simulink model "kyvadlo"  (R2017b)
settings: Solver=ode45  StartTime=0.0  StopTime=30  MaxStep=0.015  RelTol=1e-3
settings Model: Creator=ladislav  LastModifiedBy=ladislav

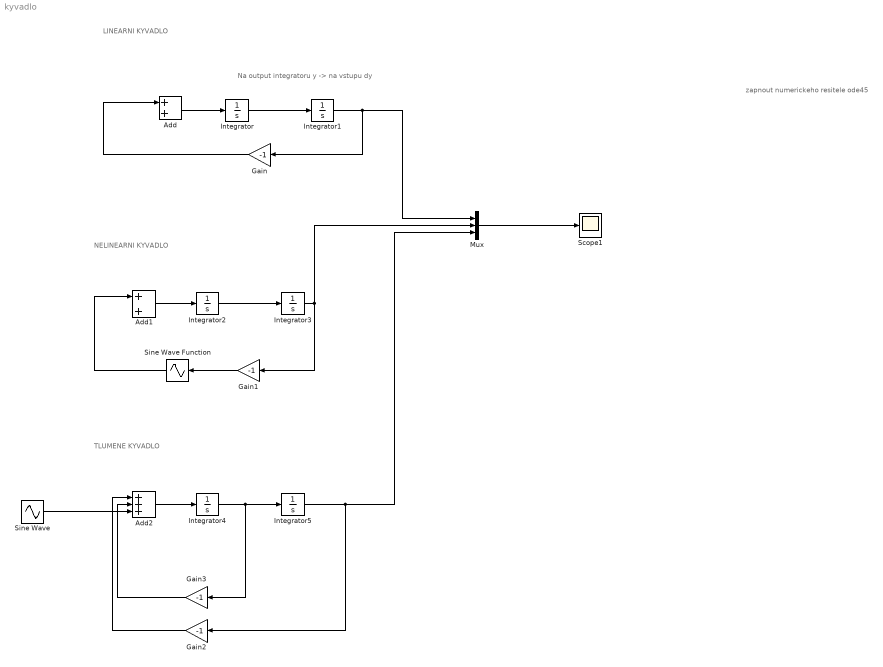
== system kyvadlo ==
  note: zapnout numerickeho resitele ode45
  note: LINEARNI KYVADLO
  note: Na output integratoru y -> na vstupu dy
  note: NELINEARNI KYVADLO
  note: TLUMENE KYVADLO
  Add : Sum
  Add1 : Sum
  Add2 : Sum  Inputs=+++
  Gain{,1..3} (4 alike) : Gain  Gain=-1
  Integrator : Integrator  InitialCondition=1.7
  Integrator1 : Integrator  InitialCondition=1
  Integrator2 : Integrator  InitialCondition=1.7
  Integrator3 : Integrator  InitialCondition=1
  Integrator4 : Integrator  InitialCondition=1.7
  Integrator5 : Integrator  InitialCondition=1
  Mux : Mux  Inputs=3
  Scope1 : Scope
  Sine Wave : Sin  Amplitude=0.2  SampleTime=0
  Sine Wave Function : Sin  TimeSource=Use external signal  SampleTime=0
  wires:
  Integrator/1 -> Integrator1/1
  Add/1 -> Integrator/1
  ? -> Add/2
  Gain/1 -> Add/1
  ? -> Add1/2
  Integrator3/1 -> Gain1/1, Mux/2
  Gain1/1 -> Sine Wave Function/1
  Integrator2/1 -> Integrator3/1
  Add1/1 -> Integrator2/1
  Sine Wave Function/1 -> Add1/1
  Mux/1 -> Scope1/1
  Integrator1/1 -> Mux/1, Gain/1
  Add2/1 -> Integrator4/1
  Integrator4/1 -> Gain3/1, Integrator5/1
  Gain2/1 -> Add2/1
  Sine Wave/1 -> Add2/3
  Integrator5/1 -> Gain2/1, Mux/3
  Gain3/1 -> Add2/2
